simulink model "model222c"  (R2024a)
settings: Solver=VariableStepAuto  StartTime=0.0  StopTime=10.0  RelTol=1e-3
settings Model: Creator=Xist  LastModifiedBy=Xist

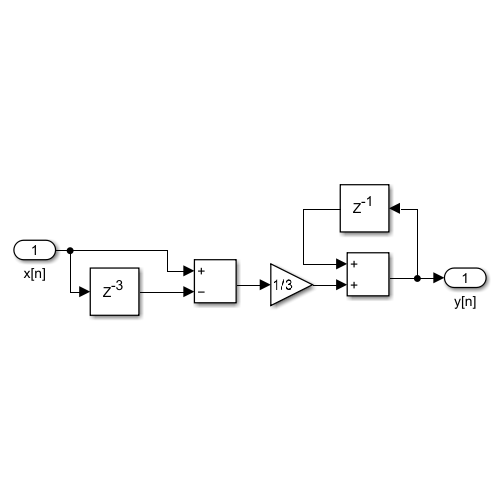
[thumbnail: Simulink's stored preview of the top-level diagram]
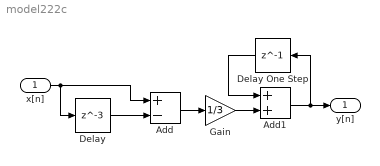
== system model222c ==
  x[n] : Inport
  Add : Sum  Inputs=+-
  Add1 : Sum
  Delay : Delay  DelayLength=3
  Delay One Step : Delay  DelayLength=1
  Gain : Gain  Gain=1/3
  y[n] : Outport
  wires:
  x[n]/1 -> Add/1, Delay/1
  Gain/1 -> Add1/2
  Delay/1 -> Add/2
  Add/1 -> Gain/1
  Delay One Step/1 -> Add1/1
  Add1/1 -> Delay One Step/1, y[n]/1
